simulink model "SimulinkExampleVelocity"  (R2022b)
settings: Solver=VariableStepAuto  StartTime=0.0  StopTime=10.0  RelTol=1e-3
undefined symbols (not defined in the file): distance0, velocity
settings Model: Creator=awolfp  LastModifiedBy=awolfp

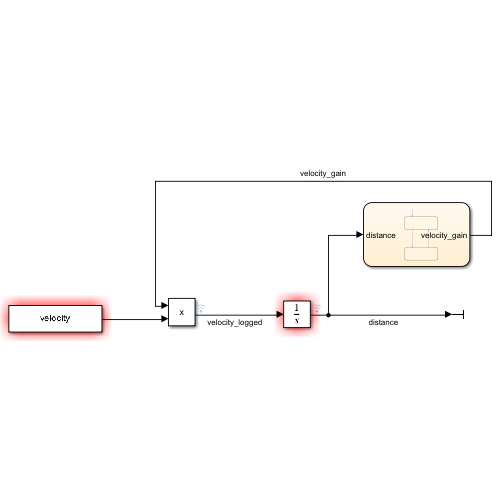
[thumbnail: Simulink's stored preview of the top-level diagram]
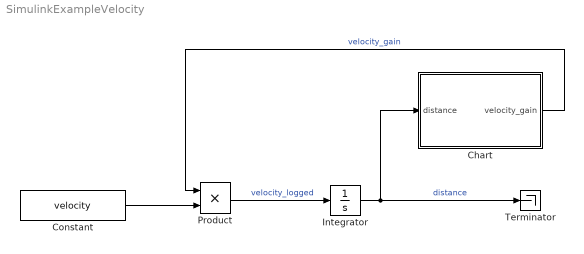
== system SimulinkExampleVelocity ==
  Chart : Stateflow chart  TreatAsAtomicUnit=on
  Constant : Constant  Value=velocity
  Integrator : Integrator  InitialCondition=distance0
  Product : Product
  Terminator : Terminator
  wires:
  Constant/1 -> Product/2
  Integrator/1 -> Chart/1(distance), Terminator/1  "distance"
  Chart/1(velocity_gain) -> Product/1  "velocity_gain"
  Product/1 -> Integrator/1  "velocity_logged"

== stateflow chart SimulinkExampleVelocity/Chart ==
  state Forward
    velocity_gain = 1;
  state Reverse
    velocity_gain = -1;
  (default) -> Forward
  Forward -> Reverse : [distance > 10]
  Reverse -> Forward : [distance < 0]
  data: distance input; velocity_gain output
